simulink model "regler_simulink"  (R2025b)
settings: Solver=FixedStepDiscrete  StartTime=0.0  StopTime=100  FixedStep=0.1  RelTol=1e-3
undefined symbols (not defined in the file): DiscIntNeverNeededParam
libraries: simulink x1
settings Model: Creator=modga  LastModifiedBy=modga

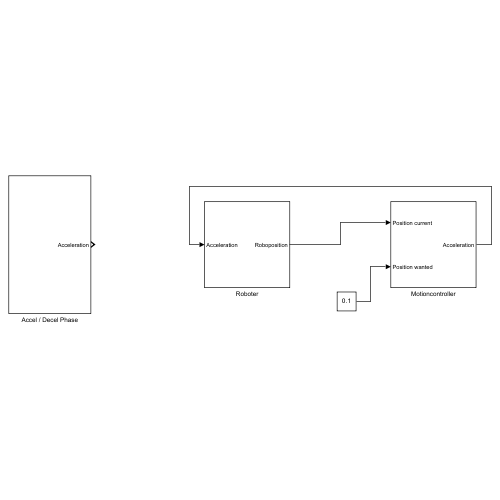
[thumbnail: Simulink's stored preview of the top-level diagram]
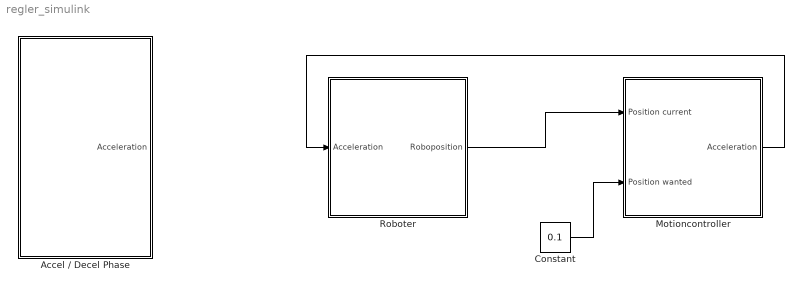
== system regler_simulink ==
  Accel / Decel Phase : Subsystem
  Constant : Constant  Value=0.1
  Motioncontroller : Subsystem
  Roboter : Subsystem
  wires:
  Constant/1 -> Motioncontroller/2(Position wanted)
  Roboter/1(Roboposition) -> Motioncontroller/1(Position current)
  Motioncontroller/1(Acceleration) -> Roboter/1(Acceleration)

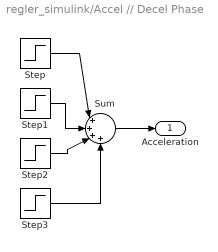
== system regler_simulink/Accel // Decel Phase ==
  Step : Step  SampleTime=0
  Step1 : Step  Time=2  After=-1  SampleTime=0
  Step2 : Step  Time=8  After=-1  SampleTime=0
  Step3 : Step  Time=9  SampleTime=0
  Sum : Sum  Inputs=|++++
  Acceleration : Outport
  wires:
  Step1/1 -> Sum/2
  Step/1 -> Sum/1
  Step2/1 -> Sum/3
  Step3/1 -> Sum/4
  Sum/1 -> Acceleration/1

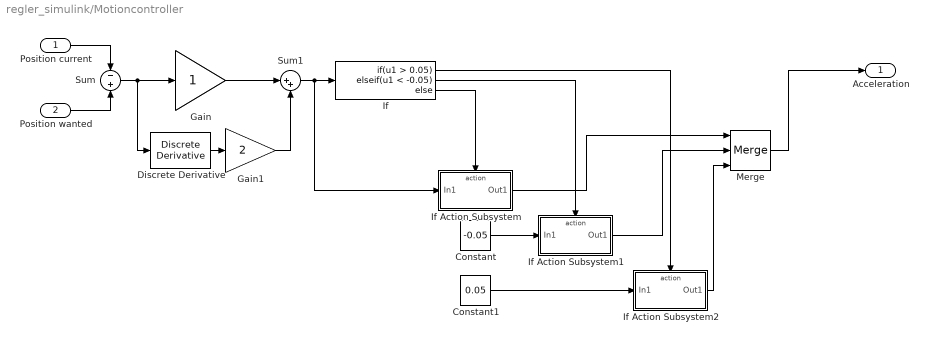
== system regler_simulink/Motioncontroller ==
  Position current : Inport
  Position wanted : Inport  Port=2
  Constant : Constant  Value=-0.05
  Constant1 : Constant  Value=0.05
  Discrete Derivative : simulink/Discrete/Discrete Derivative  gainval=1.0  ICPrevScaledInput=0.0  OutMin=[]  OutMax=[]  OutDataType=fixdt(1, 16)  OutScaling=2^-10  DoSatur=off
  Gain : Gain
  Gain1 : Gain  Gain=2
  If : If  IfExpression=u1 > 0.05  ElseIfExpressions=u1 < -0.05
  If Action Subsystem : Subsystem  TreatAsAtomicUnit=on
  If Action Subsystem1 : Subsystem  TreatAsAtomicUnit=on
  If Action Subsystem2 : Subsystem  TreatAsAtomicUnit=on
  Merge : Merge  Inputs=3
  Sum : Sum  Inputs=-+
  Sum1 : Sum  Inputs=|++
  Acceleration : Outport
  wires:
  Position wanted/1 -> Sum/2
  Sum/1 -> Discrete Derivative/1, Gain/1
  Sum1/1 -> If Action Subsystem/1(In1), If/1
  If Action Subsystem2/1(Out1) -> Merge/3
  If Action Subsystem1/1(Out1) -> Merge/2
  If Action Subsystem/1(Out1) -> Merge/1
  Constant1/1 -> If Action Subsystem2/1(In1)
  Constant/1 -> If Action Subsystem1/1(In1)
  If/3 -> If Action Subsystem/Action
  If/2 -> If Action Subsystem1/Action
  If/1 -> If Action Subsystem2/Action
  Discrete Derivative/1 -> Gain1/1
  Merge/1 -> Acceleration/1
  Position current/1 -> Sum/1
  Gain/1 -> Sum1/1
  Gain1/1 -> Sum1/2

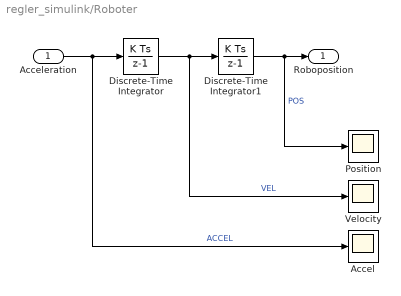
== system regler_simulink/Roboter ==
  Acceleration : Inport
  Accel : Scope
      settings: ActiveDisplayYMinimum=-0.018240092019539064  ActiveDisplayYMaximum=0.091808056779157945  DataLoggingVariableName=ScopeData2
  Discrete-Time Integrator : DiscreteIntegrator  SampleTime=0.1  ICPrevOutput=DiscIntNeverNeededParam  ICPrevScaledInput=DiscIntNeverNeededParam
  Discrete-Time Integrator1 : DiscreteIntegrator  SampleTime=0.1  ICPrevOutput=DiscIntNeverNeededParam  ICPrevScaledInput=DiscIntNeverNeededParam
  Position : Scope
      settings: ActiveDisplayYMinimum=-0.12753507389606195  ActiveDisplayYMaximum=0.4322282888788162
  Velocity : Scope
      settings: ActiveDisplayYMinimum=-0.019693384836575237  ActiveDisplayYMaximum=0.041598237464595574
  Roboposition : Outport
  wires:
  Discrete-Time Integrator1/1 -> Position/1, Roboposition/1  "POS"
  Discrete-Time Integrator/1 -> Discrete-Time Integrator1/1, Velocity/1  "VEL"
  Acceleration/1 -> Discrete-Time Integrator/1, Accel/1  "ACCEL"

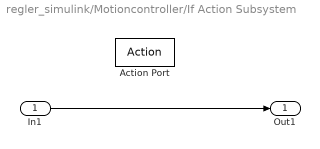
== system regler_simulink/Motioncontroller/If Action Subsystem ==
  In1 : Inport
  Action Port : ActionPort  ActionPortLabel=else
  Out1 : Outport
  wires:
  In1/1 -> Out1/1

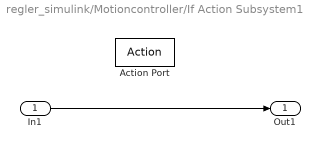
== system regler_simulink/Motioncontroller/If Action Subsystem1 ==
  In1 : Inport
  Action Port : ActionPort  ActionPortLabel=elseif(u1 < -0.05)
  Out1 : Outport
  wires:
  In1/1 -> Out1/1

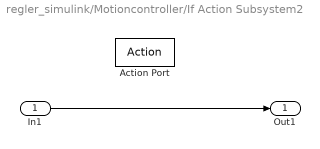
== system regler_simulink/Motioncontroller/If Action Subsystem2 ==
  In1 : Inport
  Action Port : ActionPort  ActionPortLabel=if(u1 > 0.05)
  Out1 : Outport
  wires:
  In1/1 -> Out1/1
